simulink model "Cable_Dynamics_Model_testing"  (R2019b)
settings: Solver=VariableStepAuto  StartTime=0.0  StopTime=10.0  RelTol=1e-3
values from neighbouring files (symbols this model uses):
  S = 8/1000    (= 0.008)    [parameters.m]
undefined symbols (not defined in the file or in its folder): zeta
settings Model: Creator=arund  LastModifiedBy=arund

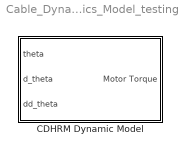
== system Cable_Dynamics_Model_testing ==
  CDHRM Dynamic Model : Subsystem

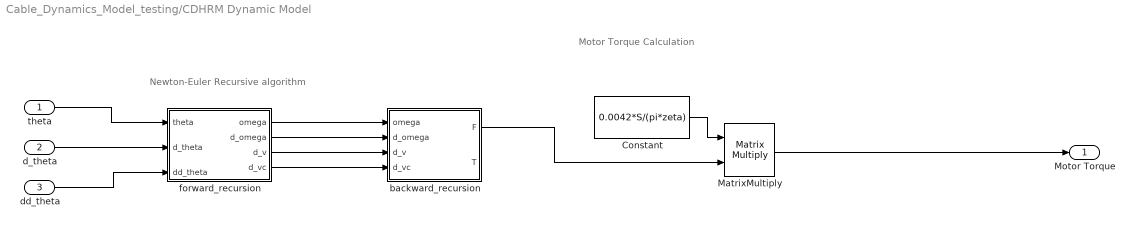
== system Cable_Dynamics_Model_testing/CDHRM Dynamic Model ==
  note: Newton-Euler Recursive algorithm
  note: Motor Torque Calculation
  theta : Inport
  d_theta : Inport  Port=2
  dd_theta : Inport  Port=3
  Constant : Constant  Value=0.0042*S/(pi*zeta)
  MatrixMultiply : Product  Multiplication=Matrix(*)
  backward_recursion : MATLAB Function  TreatAsAtomicUnit=on
  forward_recursion : MATLAB Function  TreatAsAtomicUnit=on
  Motor Torque : Outport
  wires:
  theta/1 -> forward_recursion/1(theta)
  d_theta/1 -> forward_recursion/2(d_theta)
  dd_theta/1 -> forward_recursion/3(dd_theta)
  forward_recursion/1(omega) -> backward_recursion/1(omega)
  forward_recursion/2(d_omega) -> backward_recursion/2(d_omega)
  forward_recursion/3(d_v) -> backward_recursion/3(d_v)
  forward_recursion/4(d_vc) -> backward_recursion/4(d_vc)
  backward_recursion/1(F) -> MatrixMultiply/2
  MatrixMultiply/1 -> Motor Torque/1
  Constant/1 -> MatrixMultiply/1

== matlab function Cable_Dynamics_Model_testing/CDHRM Dynamic Model/backward_recursion ==
  data: omega input; F output; d_omega input; d_v input; d_vc input; T output
function [F, T] = fcn(omega, d_omega, d_v, d_vc)

y = u;

== matlab function Cable_Dynamics_Model_testing/CDHRM Dynamic Model/forward_recursion ==
  data: theta input; omega output; d_theta input; dd_theta input; d_omega output; d_v output; d_vc output
function [omega, d_omega, d_v, d_vc] = fcn(theta, d_theta, dd_theta)
% Initial conditions
omega_1 = R_0*Z_0*d_theta(1) + R_1*Z_1*d_theta;
d_omega_1 = R_0 * (dd_theta(1))
% Initialising previous link values

y = u;
